simulink model "matlab99003728"  (R2020b)
settings: Solver=VariableStepAuto  StartTime=0.0  StopTime=20  RelTol=1e-3
undefined symbols (not defined in the file): sigbuilder_block
settings Model: Creator=99003728  LastModifiedBy=99003728

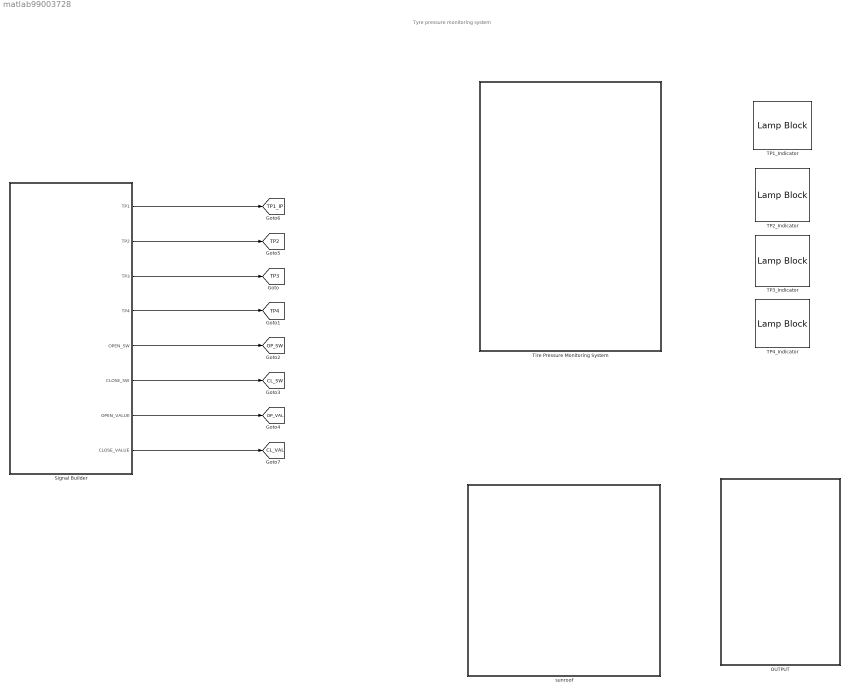
== system matlab99003728 ==
  note: Tyre pressure monitoring system
  OUTPUT : Subsystem
  Signal Builder : Subsystem  Tag=STV Subsys  LoadFcn=sigbuilder_block('load');  StartFcn=sigbuilder_block('start');  StopFcn=sigbuilder_block('stop');  ClipboardFcn=sigbuilder_block('clipboard');  mask(Sigbuilder block){tuvar=[0:10]}
      mask help: Simulink:masks:SigbuilderBlock_MD
      mask init:
      | if ~strcmp(get_param(bdroot(gcbh),'SimulationStatus'),'stopped') tuvar = sigbuilder_block('maskInit'); end
      settings: CopyFcn=sigbuilder_block('copy');  DeleteFcn=sigbuilder_block('delete');  ModelCloseFcn=sigbuilder_block('modelClose');  PreSaveFcn=sigbuilder_block('preSave');  PauseFcn=sigbuilder_block('pause');  ContinueFcn=sigbuilder_block('continue');  NameChangeFcn=sigbuilder_block('namechange');  OpenFcn=sigbuilder_block('open',[0 30 1200 587.25 ]);  CloseFcn=sigbuilder_block('close');
      mask Display: plot(0, 0, 100, 100,[2, 2, 32, 32, 2], [68, 8, 8, 68, 68],[32, 2], [38, 38], [32, 19, 2],[53, 60, 44], [32, 17, 17, 2],[16, 16, 31, 31]);txt = getActiveGroup(gcbh);text(2, 100, txt,'verticalAlignment', 'top');
  TP1_Indicator : LampBlock
  TP2_Indicator : LampBlock
  TP3_Indicator : LampBlock
  TP4_Indicator : LampBlock
  Tire Pressure Monitoring System : Subsystem
  sunroof : Subsystem
  tag scope: CL_SW=global, CL_VAL=global, OP_SW=global, OP_VAL=global, TP1_IP=global, TP2=global, TP3=global, TP4=global
  wires:
  Signal Builder/1(TP1) -> [TP1_IP]
  Signal Builder/2(TP2) -> [TP2]
  Signal Builder/3(TP3) -> [TP3]
  Signal Builder/4(TP4) -> [TP4]
  Signal Builder/5(OPEN_SW) -> [OP_SW]
  Signal Builder/6(CLOSE_SW) -> [CL_SW]
  Signal Builder/7(OPEN_VALUE) -> [OP_VAL]
  Signal Builder/8(CLOSE_VALUE) -> [CL_VAL]

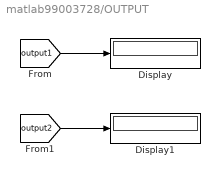
== system matlab99003728/OUTPUT ==
  Display : Display
  Display1 : Display
  wires:
  [output2] -> Display1/1
  [output1] -> Display/1

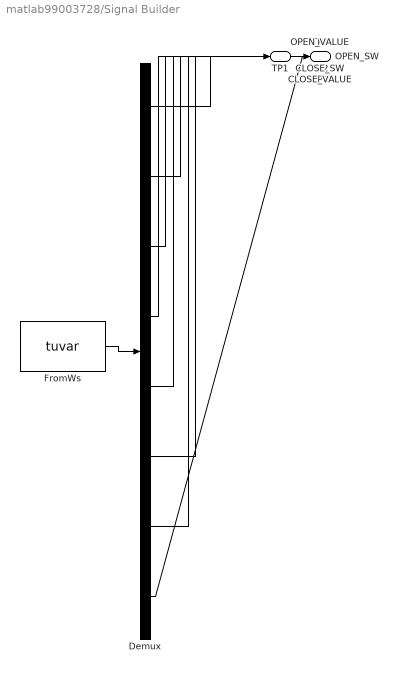
== system matlab99003728/Signal Builder ==
  Demux : Demux  Tag=STV Demux  Outputs=8
      settings: DisplayOption=none
  FromWs : FromWorkspace  Tag=STV FromWs  VariableName=tuvar  SampleTime=1
      SigBuilderData=|
      | common.afterFinalStr = 'Extrapolate'
      | common.sampleTime = '1'
      | dataSet.timeRange = [0 14]
      | dataSet.name = 'Sheet1'
      | sbobj.Name = 'Signal Builder'
      | sbobj.Groups.Name = 'Sheet1'
      | sbobj.Groups.Signals(1).Name = 'TP1'
      | sbobj.Groups.Signals(1).XData = [0 1 2 3 4 5 6 7 8 9 10 11 12 13 14]
      | sbobj.Groups.Signals(1).YData = [76 40 12 45 30 78 72 80 0 85 99 90 14 77 96]
      | sbobj.Groups.Signals(2).Name = 'TP2'
      | sbobj.Groups.Signals(2).XData = [0 1 2 3 4 5 6 7 8 9 10 11 12 13 14]
      | sbobj.Groups.Signals(2).YData = [76 40 96 45 30 78 72 80 0 85 99 90 14 77 96]
      | sbobj.Groups.Signals(3).Name = 'TP3'
      | sbobj.Groups.Signals(3).XData = [0 1 2 3 4 5 6 7 8 9 10 11 12 13 14]
      | sbobj.Groups.Signals(3).YData = [76 40 12 89 30 78 72 80 0 85 99 90 14 77 96]
      | sbobj.Groups.Signals(4).Name = 'TP4'
      | sbobj.Groups.Signals(4).XData = [0 1 2 3 4 5 6 7 8 9 10 11 12 13 14]
      | sbobj.Groups.Signals(4).YData = [76 80 82 45 1 78 72 80 0 85 99 90 14 77 96]
      | sbobj.Groups.Signals(5).Name = 'OPEN_SW'
      | sbobj.Groups.Signals(5).XData = [0 1 2 3 4 5 6 7 8 9 10 11 12 13 14]
      | sbobj.Groups.Signals(5).YData = [0 0 0 0 0 0 0 0 1 1 1 1 1 1 1]
      | sbobj.Groups.Signals(6).Name = 'CLOSE_SW'
      | sbobj.Groups.Signals(6).XData = [0 1 2 3 4 5 6 7 8 9 10 11 12 13 14]
      | sbobj.Groups.Signals(6).YData = [1 0 1 1 1 1 1 1 1 0 0 0 0 0 0]
      | sbobj.Groups.Signals(7).Name = 'OPEN_VALUE'
      | sbobj.Groups.Signals(7).XData = [0 1 2 3 4 5 6 7 8 9 10 11 12 13 14]
      | sbobj.Groups.Signals(7).YData = [76 40 12 45 30 78 72 80 0 85 99 90 14 77 96]
      | sbobj.Groups.Signals(8).Name = 'CLOSE_VALUE'
      | sbobj.Groups.Signals(8).XData = [0 1 2 3 4 5 6 7 8 9 10 11 12 13 14]
      | sbobj.Groups.Signals(8).YData = [76 40 12 45 30 78 72 80 0 85 99 90 14 77 96]
      | sbobj.Groups.TimeRange = [0 14]
  TP1 : Outport  Tag=STV Outport
  TP2 : Outport  Tag=STV Outport  Port=2
  TP3 : Outport  Tag=STV Outport  Port=3
  TP4 : Outport  Tag=STV Outport  Port=4
  OPEN_SW : Outport  Tag=STV Outport  Port=5
  CLOSE_SW : Outport  Tag=STV Outport  Port=6
  OPEN_VALUE : Outport  Tag=STV Outport  Port=7
  CLOSE_VALUE : Outport  Tag=STV Outport  Port=8
  wires:
  Demux/1 -> TP1/1
  FromWs/1 -> Demux/1
  Demux/2 -> TP2/1
  Demux/3 -> TP3/1
  Demux/4 -> TP4/1
  Demux/5 -> OPEN_SW/1
  Demux/6 -> CLOSE_SW/1
  Demux/7 -> OPEN_VALUE/1
  Demux/8 -> CLOSE_VALUE/1

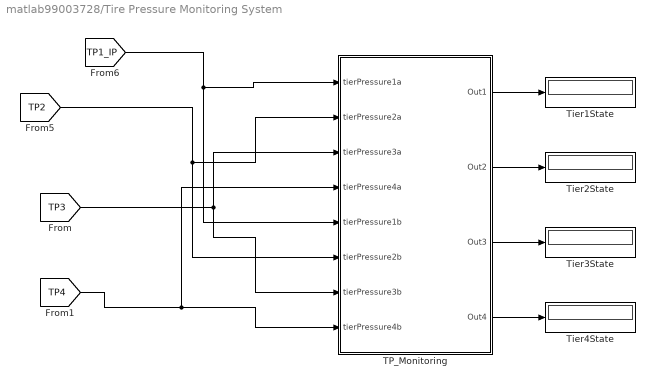
== system matlab99003728/Tire Pressure Monitoring System ==
  TP_Monitoring : Subsystem
  Tier1State : Display
  Tier2State : Display
  Tier3State : Display
  Tier4State : Display
  wires:
  TP_Monitoring/2(Out2) -> Tier2State/1
  [TP4] -> TP_Monitoring/4(tierPressure4a), TP_Monitoring/8(tierPressure4b)
  TP_Monitoring/1(Out1) -> Tier1State/1
  [TP1_IP] -> TP_Monitoring/1(tierPressure1a), TP_Monitoring/5(tierPressure1b)
  [TP3] -> TP_Monitoring/7(tierPressure3b), TP_Monitoring/3(tierPressure3a)
  TP_Monitoring/3(Out3) -> Tier3State/1
  [TP2] -> TP_Monitoring/6(tierPressure2b), TP_Monitoring/2(tierPressure2a)
  TP_Monitoring/4(Out4) -> Tier4State/1

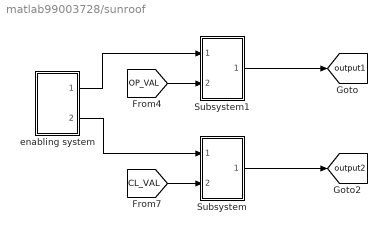
== system matlab99003728/sunroof ==
  Subsystem : Subsystem
  Subsystem1 : Subsystem
  enabling system : Subsystem
  tag scope: output1=global, output2=global
  wires:
  enabling system/1(Outport) -> Subsystem1/1(Enable)
  enabling system/2(enableO) -> Subsystem/1(Enable)
  [CL_VAL] -> Subsystem/2(Inport)
  [OP_VAL] -> Subsystem1/2(Inport)
  Subsystem/1(Outport) -> [output2]
  Subsystem1/1(Outport) -> [output1]

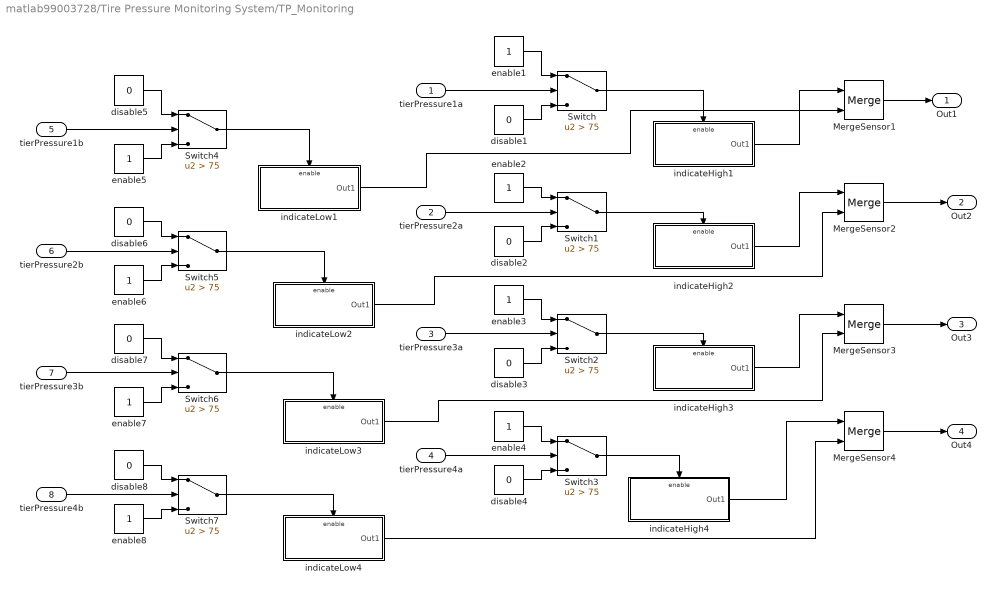
== system matlab99003728/Tire Pressure Monitoring System/TP_Monitoring ==
  tierPressure1a : Inport
  tierPressure2a : Inport  Port=2
  tierPressure3a : Inport  Port=3
  tierPressure4a : Inport  Port=4
  tierPressure1b : Inport  Port=5
  tierPressure2b : Inport  Port=6
  tierPressure3b : Inport  Port=7
  tierPressure4b : Inport  Port=8
  MergeSensor{1..4} (4 alike) : Merge
  Switch{,1..7} (8 alike) : Switch  Criteria=u2 > Threshold  Threshold=75
  disable{1..8} (8 alike) : Constant  Value=0
  enable{1..8} (8 alike) : Constant
  indicateHigh1 : Subsystem  TreatAsAtomicUnit=on
  indicateHigh2 : Subsystem  TreatAsAtomicUnit=on
  indicateHigh3 : Subsystem  TreatAsAtomicUnit=on
  indicateHigh4 : Subsystem  TreatAsAtomicUnit=on
  indicateLow1 : Subsystem  TreatAsAtomicUnit=on
  indicateLow2 : Subsystem  TreatAsAtomicUnit=on
  indicateLow3 : Subsystem  TreatAsAtomicUnit=on
  indicateLow4 : Subsystem  TreatAsAtomicUnit=on
  Out1 : Outport
  Out2 : Outport  Port=2
  Out3 : Outport  Port=3
  Out4 : Outport  Port=4
  wires:
  enable1/1 -> Switch/1
  tierPressure3a/1 -> Switch2/2
  disable1/1 -> Switch/3
  disable3/1 -> Switch2/3
  enable2/1 -> Switch1/1
  tierPressure1a/1 -> Switch/2
  disable4/1 -> Switch3/3
  disable2/1 -> Switch1/3
  enable4/1 -> Switch3/1
  tierPressure2a/1 -> Switch1/2
  tierPressure4a/1 -> Switch3/2
  enable3/1 -> Switch2/1
  disable8/1 -> Switch7/1
  enable8/1 -> Switch7/3
  disable6/1 -> Switch5/1
  enable6/1 -> Switch5/3
  enable7/1 -> Switch6/3
  enable5/1 -> Switch4/3
  disable5/1 -> Switch4/1
  tierPressure2b/1 -> Switch5/2
  tierPressure3b/1 -> Switch6/2
  tierPressure1b/1 -> Switch4/2
  disable7/1 -> Switch6/1
  tierPressure4b/1 -> Switch7/2
  MergeSensor1/1 -> Out1/1
  MergeSensor2/1 -> Out2/1
  MergeSensor3/1 -> Out3/1
  MergeSensor4/1 -> Out4/1
  Switch3/1 -> indicateHigh4/Enable
  Switch2/1 -> indicateHigh3/Enable
  Switch1/1 -> indicateHigh2/Enable
  Switch/1 -> indicateHigh1/Enable
  Switch7/1 -> indicateLow4/Enable
  Switch6/1 -> indicateLow3/Enable
  Switch5/1 -> indicateLow2/Enable
  Switch4/1 -> indicateLow1/Enable
  indicateHigh1/1(Out1) -> MergeSensor1/1
  indicateLow1/1(Out1) -> MergeSensor1/2
  indicateHigh2/1(Out1) -> MergeSensor2/1
  indicateLow2/1(Out1) -> MergeSensor2/2
  indicateHigh3/1(Out1) -> MergeSensor3/1
  indicateLow3/1(Out1) -> MergeSensor3/2
  indicateHigh4/1(Out1) -> MergeSensor4/1
  indicateLow4/1(Out1) -> MergeSensor4/2

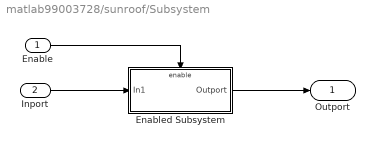
== system matlab99003728/sunroof/Subsystem ==
  Enable : Inport
  Inport : Inport  Port=2
  Enabled Subsystem : Subsystem  TreatAsAtomicUnit=on
  Outport : Outport
  wires:
  Enabled Subsystem/1(Outport) -> Outport/1
  Inport/1 -> Enabled Subsystem/1(In1)
  Enable/1 -> Enabled Subsystem/Enable

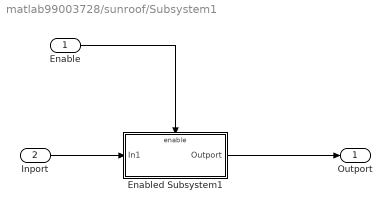
== system matlab99003728/sunroof/Subsystem1 ==
  Enable : Inport
  Inport : Inport  Port=2
  Enabled Subsystem1 : Subsystem  TreatAsAtomicUnit=on
  Outport : Outport
  wires:
  Inport/1 -> Enabled Subsystem1/1(In1)
  Enabled Subsystem1/1(Outport) -> Outport/1
  Enable/1 -> Enabled Subsystem1/Enable

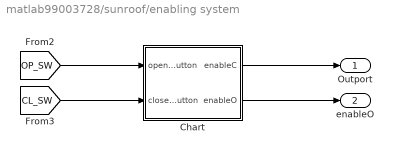
== system matlab99003728/sunroof/enabling system ==
  Chart : Stateflow chart  TreatAsAtomicUnit=on
      settings: PortSchema="{\"entries\":[{\"content\":{\"sides\":[{\"content\":{\"connectorIds\":[\"In2\",\"In1\"]},\"type\":\"ConnectorPlacement.EquallySpacedRectSide\",\"uuid\":\"e77fb548-5411-4dff-a09c-dcff2e4e83fa\"},{\"content\":{\"connectorIds\":[\"Out1\",\"Out2\"],\"side\":\"RIGHT\"},\"type\":\"ConnectorPlacement.EquallySpacedRectSide\",\"uuid\":\"fb2d12f5-730f-4265-a3f8-30409b75040e\"},{\"content\":{\"connectorIds\":[],\"side\":\"TOP\"},\"type\":\"ConnectorPlacement.EquallySpacedRectSide\",\"uuid\":\"5ec706c6-4a0b-4294-a183-09121d2d4adc\"},{\"content\":{\"connectorIds\":[],\"side\":\"HIDDEN\"},\"type\":\"ConnectorPlacement.EquallySpacedRectSide\",\"uuid\":\"e64ccab7-f9d3-41b0-81fa-c7461dca4746\"}]},\"type\":\"ConnectorPlacement.EquallySpacedConnector\",\"uuid\":\"e8c87857-404b-4a97-9417-fff31936aad1\"}],\"packageUris\":[\"http://schema.mathworks.com/mf0/Connector/R2020b\"],\"version\":\"1.0\"}"
  Outport : Outport
  enableO : Outport  Port=2
  wires:
  Chart/1(enableC) -> Outport/1
  [CL_SW] -> Chart/1(closeButton)
  Chart/2(enableO) -> enableO/1
  [OP_SW] -> Chart/2(openButton)

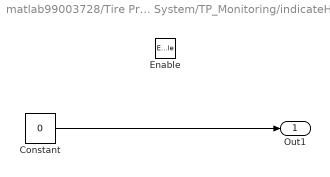
== system matlab99003728/Tire Pressure Monitoring System/TP_Monitoring/indicateHigh1 ==
  Enable : EnablePort
  Constant : Constant  Value=0
  Out1 : Outport
  wires:
  Constant/1 -> Out1/1

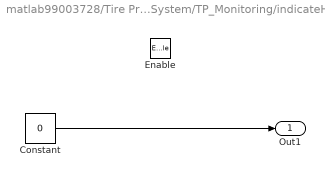
== system matlab99003728/Tire Pressure Monitoring System/TP_Monitoring/indicateHigh2 ==
  Enable : EnablePort
  Constant : Constant  Value=0
  Out1 : Outport
  wires:
  Constant/1 -> Out1/1

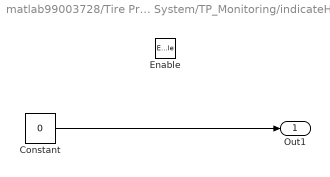
== system matlab99003728/Tire Pressure Monitoring System/TP_Monitoring/indicateHigh3 ==
  Enable : EnablePort
  Constant : Constant  Value=0
  Out1 : Outport
  wires:
  Constant/1 -> Out1/1

== system matlab99003728/Tire Pressure Monitoring System/TP_Monitoring/indicateHigh4 ==
  Enable : EnablePort
  Constant : Constant  Value=0
  Out1 : Outport
  wires:
  Constant/1 -> Out1/1

== system matlab99003728/Tire Pressure Monitoring System/TP_Monitoring/indicateLow1 ==
  Enable : EnablePort
  Constant : Constant
  Out1 : Outport
  wires:
  Constant/1 -> Out1/1

== system matlab99003728/Tire Pressure Monitoring System/TP_Monitoring/indicateLow2 ==
  Enable : EnablePort
  Constant : Constant
  Out1 : Outport
  wires:
  Constant/1 -> Out1/1

== system matlab99003728/Tire Pressure Monitoring System/TP_Monitoring/indicateLow3 ==
  Enable : EnablePort
  Constant : Constant
  Out1 : Outport
  wires:
  Constant/1 -> Out1/1

== system matlab99003728/Tire Pressure Monitoring System/TP_Monitoring/indicateLow4 ==
  Enable : EnablePort
  Constant : Constant
  Out1 : Outport
  wires:
  Constant/1 -> Out1/1

== system matlab99003728/sunroof/Subsystem/Enabled Subsystem ==
  In1 : Inport
  Enable : EnablePort
  Outport : Outport
  wires:
  In1/1 -> Outport/1

== system matlab99003728/sunroof/Subsystem1/Enabled Subsystem1 ==
  In1 : Inport
  Enable : EnablePort
  Outport : Outport
  wires:
  In1/1 -> Outport/1

== stateflow chart matlab99003728/sunroof/enabling system/Chart ==
  state stage1
    entry:
    enableO=0;
    enableC=0;
  state stage3
    entry:
    enableO=1;
    enableC=0;
  state stage2
    entry:
    enableO=0;
    enableC=1;
  (default) -> stage1
  stage1 -> stage3 [order 3] : [openButton ==1 && closeButton==0]
  stage1 -> stage2 [order 1] : [openButton ==0 && closeButton==1]
  stage2 -> stage1 : [(openButton ==1 && closeButton==1) || (openButton ==0 && closeButton==0)]
  stage3 -> stage1 : [(openButton ==1 && closeButton==1) || (openButton ==0 && closeButton==0)]
  stage1 -> stage1 [order 2] : [(openButton ==1 && closeButton==1) || (openButton ==0 && closeButton==0)]
  data: closeButton input; openButton input; enableC output; enableO output
